simulink model "pendulum_core"  (R2024b)
settings: Solver=ode1  StartTime=0.0  StopTime=5  FixedStep=0.01  MaxStep=0.001  RelTol=1e-3
settings Model: Creator=mattf  LastModifiedBy=benva
settings DataIOCC: SaveFinalState=on  SaveOperatingPoint=on  SaveFormat=Array  SaveOutput=off  ReturnWorkspaceOutputs=off

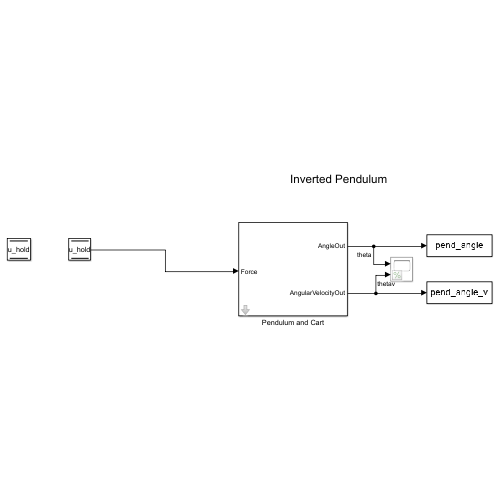
[thumbnail: Simulink's stored preview of the top-level diagram]
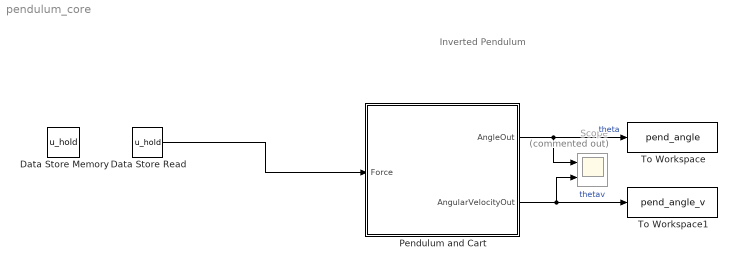
== system pendulum_core ==
  note: Inverted Pendulum
  Data Store Memory : DataStoreMemory  DataStoreName=u_hold  WriteAfterWriteMsg=warning  ShowAdditionalParam=off
  Data Store Read : DataStoreRead  DataStoreName=u_hold  IndexOptions=Index vector (dialog)  Indices=1  OutputSizes=1
  Pendulum and Cart : Subsystem  mask{m=0.2, l=0.3/2, g=9.8, init=0.07}
      mask prompts: m "Pend Mass (kg):"; l "COM Distance (m):"; g "Acc due to Gravity (g):"; init "Initial Angle (rad):"
  Scope : Scope  Commented=on  NumInputPorts=2
  To Workspace : ToWorkspace  VariableName=pend_angle  SampleTime=-1
  To Workspace1 : ToWorkspace  VariableName=pend_angle_v  SampleTime=-1
  wires:
  Pendulum and Cart/1(AngleOut) -> To Workspace/1, Scope/1  "theta"
  Pendulum and Cart/2(AngularVelocityOut) -> Scope/2, To Workspace1/1  "thetav"
  Data Store Read/1 -> Pendulum and Cart/1(Force)

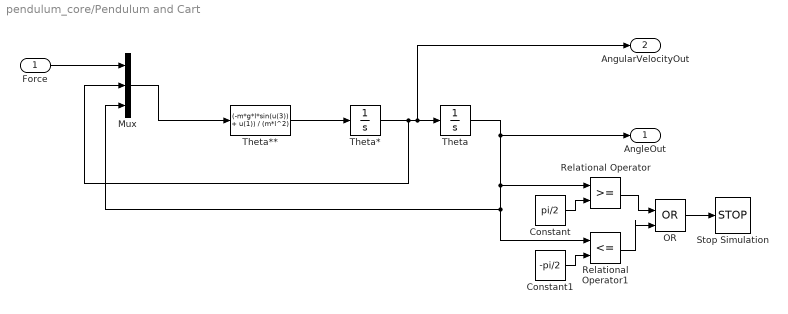
== system pendulum_core/Pendulum and Cart ==
  Force : Inport
  Constant : Constant  Value=pi/2
  Constant1 : Constant  Value=-pi/2
  Mux : Mux  Inputs=3
  OR : Logic  Operator=OR  IconShape=distinctive  AllPortsSameDT=off  OutDataTypeStr=boolean
  Relational Operator : RelationalOperator  OutDataTypeStr=boolean  RndMeth=Simplest  InputSameDT=off
  Relational Operator1 : RelationalOperator  Operator=<=  OutDataTypeStr=boolean  RndMeth=Simplest  InputSameDT=off
  Stop Simulation : Stop
  Theta : Integrator  InitialCondition=init
  Theta* : Integrator
  Theta** : Fcn  Expr=(-m*g*l*sin(u(3)) + u(1)) / (m*l^2)
  AngleOut : Outport
  AngularVelocityOut : Outport  Port=2
  wires:
  Mux/1 -> Theta**/1
  Force/1 -> Mux/1
  Theta**/1 -> Theta*/1
  Theta/1 -> AngleOut/1, Relational Operator1/1, Mux/3, Relational Operator/1
  Theta*/1 -> Mux/2, AngularVelocityOut/1, Theta/1
  Constant/1 -> Relational Operator/2
  OR/1 -> Stop Simulation/1
  Relational Operator1/1 -> OR/2
  Constant1/1 -> Relational Operator1/2
  Relational Operator/1 -> OR/1
